simulink model "Satellite"  (R2021b)
settings: Solver=VariableStepAuto  StartTime=0.0  StopTime=10.0  RelTol=1e-3
settings Model: Creator=DELL  LastModifiedBy=DELL

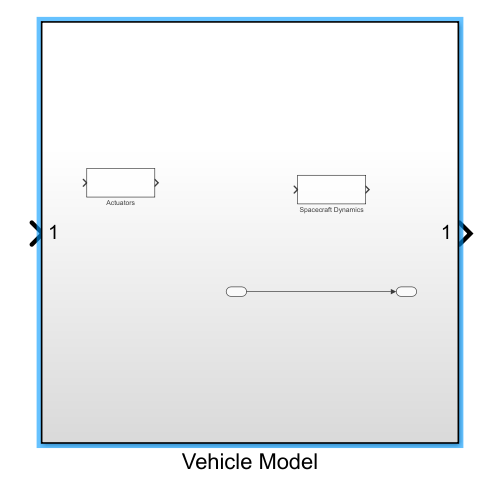
[thumbnail: Simulink's stored preview of the top-level diagram]
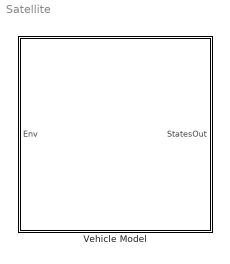
== system Satellite ==
  Vehicle Model : Subsystem

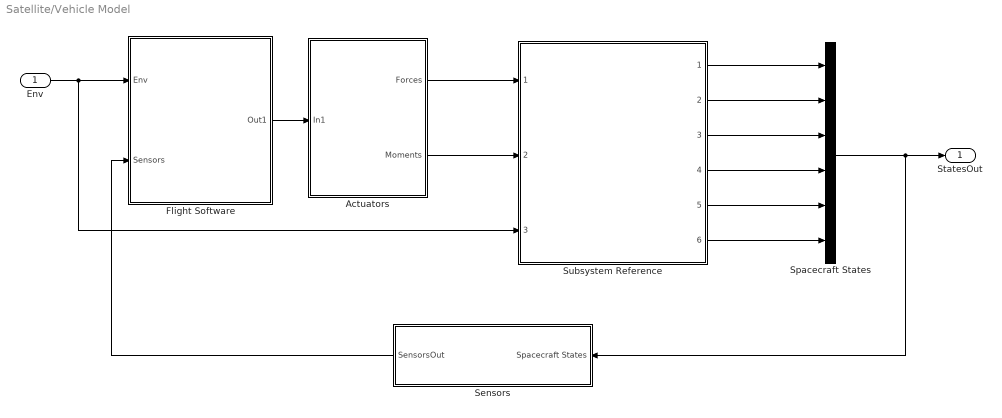
== system Satellite/Vehicle Model ==
  Env : Inport
  Actuators : Subsystem
  Flight Software : Subsystem
  Sensors : Subsystem
  Spacecraft States : Mux  Inputs=6
  Subsystem Reference : Subsystem  ReferencedSubsystem=Spacecraft_Dynamics  Mass=1  J=eye(3)
  StatesOut : Outport
  wires:
  Flight Software/1(Out1) -> Actuators/1(In1)
  Env/1 -> Subsystem Reference/3, Flight Software/1(Env)
  Subsystem Reference/1 -> Spacecraft States/1
  Spacecraft States/1 -> Sensors/1(Spacecraft States), StatesOut/1
  Sensors/1(SensorsOut) -> Flight Software/2(Sensors)
  Subsystem Reference/2 -> Spacecraft States/2
  Subsystem Reference/3 -> Spacecraft States/3
  Subsystem Reference/4 -> Spacecraft States/4
  Subsystem Reference/5 -> Spacecraft States/5
  Subsystem Reference/6 -> Spacecraft States/6
  Actuators/2(Moments) -> Subsystem Reference/2
  Actuators/1(Forces) -> Subsystem Reference/1

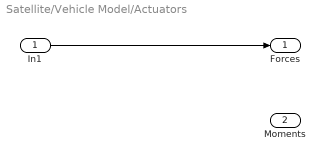
== system Satellite/Vehicle Model/Actuators ==
  In1 : Inport
  Forces : Outport
  Moments : Outport  Port=2
  wires:
  In1/1 -> Forces/1

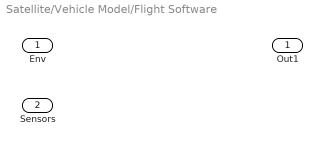
== system Satellite/Vehicle Model/Flight Software ==
  Env : Inport
  Sensors : Inport  Port=2
  Out1 : Outport

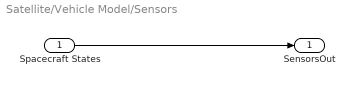
== system Satellite/Vehicle Model/Sensors ==
  Spacecraft States : Inport
  SensorsOut : Outport
  wires:
  Spacecraft States/1 -> SensorsOut/1
